simulink model "BATTERY_PV_IMPLEMENTATION"  (R2024a)
settings: Solver=VariableStepAuto  StartTime=0.0  StopTime=0.23  RelTol=1e-3
values from neighbouring files (symbols this model uses):
  a = 1.3    [TEST.m]    (also in batter_y.m = -k_omega / J)
  beta = [0.0000, 0.0306, 0.0560, 0.0772, 0.0953, 0.1113, 0.1254, 0.1382,          0.1499, 0.1607, 0.1783, 0.2134, 0.2421, 0.2669, 0.2890, 0.3091,          0.3279, 0.3456, 0.3625, 0.3789]'    [batter_y.m]
  Cdc = 278e-3    (= 0.278)    [TEST.m]    (also in batter_y.m)
  Clink = 2 * (3 / 4) * (Pnom / Fnom * 2 / Vnom_dc^2)    (= 0.325520833333)    [batter_y.m]
  fg = 60    [TEST.m]    (also in batter_y.m)
  Fnom = 60    [batter_y.m]
  Gn = 1000    [TEST.m]    (also in batter_y.m)
  Ipv_n = Isc_n*(Rp+Rs)/Rp    (= 8.21426513558)    [TEST.m]    (also in batter_y.m)
  Isc_n = 8.21    [TEST.m]    (also in batter_y.m)
  k = 1.3806503e-23    [TEST.m]    (also in batter_y.m)
  k_I = a./(b.*tau_ref)    [batter_y.m]
  k_P = 5./(b.*tau_ref)    [batter_y.m]
  KI = 0.0032    [TEST.m]    (also in batter_y.m)
  Ki_C = Rc/tau_C    (= 0.768)    [TEST.m]    (also in batter_y.m)
  Ki_DC = omega_DC^2*Cdc    [TEST.m]    (also in batter_y.m)
  Ki_Ireg = 20    [batter_y.m]
  Ki_P = 1/(Ki_pq*tau_P)    [TEST.m]    (also in batter_y.m)
  Ki_PLL = Kp_PLL/tau_PLL    [TEST.m]    (also in batter_y.m)
  Kp_C = Lc/tau_C    (= 0.020372)    [TEST.m]    (also in batter_y.m)
  Kp_DC = 2*xi_DC*omega_DC*Cdc    [TEST.m]    (also in batter_y.m)
  Kp_Ireg = 0.3    [batter_y.m]
  Kp_P = tau_C/(Ki_pq*tau_P)    [TEST.m]    (also in batter_y.m)
  Kp_PLL = xi_PLL*2*omega_PLL/Vp    [TEST.m]    (also in batter_y.m)
  KV = -0.123    [TEST.m]    (also in batter_y.m)
  KVmp = Vmp_n/Voc_n    (= 0.799392097264)    [TEST.m]    (also in batter_y.m)
  Lc = 20.372e-6    (= 2.0372e-05)    [TEST.m]    (also in batter_y.m)
  Lchoke = 0.15    [batter_y.m]
  Ltot_pu = Lxf + Lchoke    (= 0.21)    [batter_y.m]
  Lxf = TotalLeakage    (= 0.06)    [batter_y.m]
  Np = 345    [TEST.m]    (also in batter_y.m)
  Ns = 45    [TEST.m]    (also in batter_y.m)
  Ns_cell = 54    [TEST.m]    (also in batter_y.m)
  Pnom = PnomkW*1e3    (= 500000)    [TEST.m]    (also in batter_y.m = 1500000)
  q = 1.6021764e-19    [TEST.m]    (also in batter_y.m)
  Rc = 0.768e-3    (= 0.000768)    [TEST.m]    (also in batter_y.m)
  Rchoke = 0.15 / 100    (= 0.0015)    [batter_y.m]
  Rp = 425.405    [TEST.m]    (also in batter_y.m)
  Rs = 0.221    [TEST.m]    (also in batter_y.m)
  Rtot_pu = Rxf + Rchoke    (= 0.0039)    [batter_y.m]
  Rxf = TotalLeakage / 25    (= 0.0024)    [batter_y.m]
  Tn = 25    [TEST.m]    (also in batter_y.m)
  Ts = 5e-5    (= 5e-05)    [TEST.m]    (also in batter_y.m)
  Ts_Control = 5e-5    (= 5e-05)    [TEST.m]    (also in batter_y.m)
  v = [11.2600, 11.5378, 11.8156, 12.0933, 12.3711, 12.6489, 12.9267,       13.2044, 13.4822, 13.7600, 14.2600, 15.4533, 16.6467, 17.8400,       19.0333, 20.2267, 21.4200, 22.6133, 23.8067, 25.0000]'    [batter_y.m]
  Vdc = 1200    [TEST.m]    (also in batter_y.m)
  Vnom_dc = 480    [batter_y.m]
  Vnom_prim = 2400    [batter_y.m]
  Vnom_sec = 0.85 * Vnom_dc / 2 / sqrt(2) * sqrt(3)    [batter_y.m]
  Voc_n = 32.9    [TEST.m]    (also in batter_y.m)
  Vp = Ug*sqrt(2)/sqrt(3)    [TEST.m]    (also in batter_y.m)
  Zbase = Vnom_sec^2 / Pnom    [batter_y.m]
undefined symbols (not defined in the file or in its folder): D1, Delta, Ion, Lithium, para_mdl
libraries: spsSeriesRLCBranchLib x25, slpidlib x11, spsThreePhaseSeriesRLCLoadLib x9, spsThreePhaseVIMeasurementLib x7, spsSeriesRLCLoadLib x5, spsGroundLib x5, spsThreePhaseTransformerTwoWindingsLib x5, spsabctodq0Lib x4, spsControlledVoltageSourceLib x3, spsPower3phInstantaneousLib x3, spsCurrentMeasurementLib x2, spsControlledCurrentSourceLib x2
(part 3 of 3)

== system BATTERY_PV_IMPLEMENTATION/Subsystem2/Current Control/Current Regulator ==
  note: Id positive --> The converter generates active power ("Inverter mode") = Active Power P positive
  note: Iq positive --> The converter absorbs reactive power ("Inductive mode") = Reactive Power Q negative
  note: Sign Convention: Current going out of the converter = positive current
  note: Current Regulator
      | ================
  VdVq_meas : Inport  PortDimensions=2
  IdIq_meas : Inport  Port=2  PortDimensions=2
  IdIq_ref : Inport  Port=3  PortDimensions=2
  Add1 : Sum  Inputs=++-
  Add2 : Sum
  Add3 : Sum  Inputs=+++
  Demux : Demux  Outputs=2
  Demux1 : Demux  Outputs=2
  Lff : Gain  Gain=Ltot_pu  SaturateOnIntegerOverflow=on  OutDataTypeStr=Inherit: Same as input  ParamDataTypeStr=Inherit: Same as input
  "Lff  " : Gain  Gain=Ltot_pu  SaturateOnIntegerOverflow=on  OutDataTypeStr=Inherit: Same as input  ParamDataTypeStr=Inherit: Same as input
  Mux : Mux  Inputs=2
  PI : slpidlib/PID Controller  Controller=PI  Form=Parallel  TimeDomain=Discrete-time  UseExternalTs=off  SampleTime=Ts_Control  IntegratorMethod=Forward Euler  FilterMethod=Forward Euler  ControllerParametersSource=internal  P=Kp_Ireg  I=Ki_Ireg  UseKiTs=off  D=0  UseExternalDerivativeSource=off  N=100  UseFilter=on  TunerSelectOption=Transfer Function Based (PID Tuner App)  InitialConditionSource=internal  InitialConditionForIntegrator=0  InitialConditionForFilter=0  DifferentiatorICPrevScaledInput=0  ExternalReset=none  TrackingMode=off  Kt=1  LimitOutput=on  SatLimitsSource=internal  UpperSaturationLimit=1.5  LowerSaturationLimit=-1.5  LinearizeAsGain=off  AntiWindupMode=clamping  Kb=1  LimitIntegrator=off  UpperIntegratorSaturationLimit=inf  LowerIntegratorSaturationLimit=-inf  POutMin=[]  POutMax=[]  IOutMin=[]  IOutMax=[]  DOutMin=[]  DOutMax=[]  NOutMin=[]  NOutMax=[]  SumOutMin=[]  SumOutMax=[]  SaturationOutMin=[]  SaturationOutMax=[]  PParamMin=[]  PParamMax=[]  IParamMin=[]  IParamMax=[]  DParamMin=[]  DParamMax=[]  NParamMin=[]  NParamMax=[]  KbParamMin=[]  KbParamMax=[]  KtParamMin=[]  KtParamMax=[]  KbOutMin=[]  KbOutMax=[]  KtOutMin=[]  KtOutMax=[]  IntegratorOutMin=[]  IntegratorOutMax=[]  FilterOutMin=[]  FilterOutMax=[]  SumI1OutMin=[]  SumI1OutMax=[]  SumI2OutMin=[]  SumI2OutMax=[]  SumI3OutMin=[]  SumI3OutMax=[]  SumI4OutMin=[]  SumI4OutMax=[]  SumDOutMin=[]  SumDOutMax=[]  DifferentiatorOutMin=[]  DifferentiatorOutMax=[]  FilterDiffOutCoefMin=[]  FilterDiffOutCoefMax=[]  ReciprocalOutMin=[]  ReciprocalOutMax=[]  SumDenOutMin=[]  SumDenOutMax=[]  SumNumOutMin=[]  SumNumOutMax=[]  DivideOutMin=[]  DivideOutMax=[]  UdiffTsProdOutMin=[]  UdiffTsProdOutMax=[]  NTsProdOutMin=[]  NTsProdOutMax=[]  UintegralTsProdOutMin=[]  UintegralTsProdOutMax=[]  UngainTsProdOutMin=[]  UngainTsProdOutMax=[]  ClampingZeroOutDataTypeStr=Inherit: Inherit via back propagation  ClampingZeroOutMin=[]  ClampingZeroOutMax=[]  FilterDenConstantOutDataTypeStr=Inherit: Inherit via back propagation  FilterDenConstantOutMin=[]  FilterDenConstantOutMax=[]  PCopyOutDataTypeStr=Inherit: Inherit via back propagation  PCopyOutMin=[]  PCopyOutMax=[]  NCopyOutDataTypeStr=Inherit: Inherit via back propagation  NCopyOutMin=[]  NCopyOutMax=[]  IntegratorContinuousStateAttributes=''  IntegratorStateMustResolveToSignalObject=off  IntegratorRTWStateStorageClass=Auto  FilterContinuousStateAttributes=''  FilterStateMustResolveToSignalObject=off  FilterRTWStateStorageClass=Auto  ParallelPVariant=InternalParameters  IdealPVariant=Disabled  IVariant=InternalParameters  DVariant=Disabled  IntegratorVariant=Discrete  SatVariant=Enabled  AWVariant=DiscClampingParallel  PCopyVariant=Disabled  TRVariant=Disabled  FdbkBlocksVariant=Forward  IdealPFdbkVariant=Disabled  SatFdbkVariant=Disabled  DerivativeFilterVariant=Disabled  NVariant=Disabled  NCopyVariant=Disabled_SignalSpec  FilterICVariant=Disabled  IntegratorICVariant=InternalICs  ExternalResetVariant=Disabled  TRSumVariant=Passthrough  SumFdbkVariant=Disabled  SumVariant=Sum_PI  TsampFilterVariant=InternalTs  TsampNgainVariant=Passthrough  TsampIntegralVariant=Disabled_SignalSpec  ExternalSaturationOutDataTypeStr=Inherit: Same as second input  DerivativeSourceVariant=Disabled
  Rff : Gain  Gain=Rtot_pu  SaturateOnIntegerOverflow=on  OutDataTypeStr=Inherit: Same as input  ParamDataTypeStr=Inherit: Same as input
  "Rff " : Gain  Gain=Rtot_pu  SaturateOnIntegerOverflow=on  OutDataTypeStr=Inherit: Same as input  ParamDataTypeStr=Inherit: Same as input
  Saturation : Saturate  UpperLimit=1.5  LowerLimit=-1.5
  Scope : Scope  NumInputPorts=2
  Sum : Sum  Inputs=|-+
  VdVq_conv : Outport  VectorParamsAs1DForOutWhenUnconnected=off
  wires:
  Add3/1 -> Mux/2
  Demux/2 -> Add3/1
  Add1/1 -> Mux/1  "Feedforward"
  Lff/1 -> Add3/3
  Rff/1 -> Add3/2
  Demux1/2 -> Rff/1, "Lff  "/1
  "Lff  "/1 -> Add1/3
  Demux1/1 -> Lff/1, "Rff "/1
  "Rff "/1 -> Add1/2
  Demux/1 -> Add1/1
  VdVq_meas/1 -> Demux/1
  Saturation/1 -> VdVq_conv/1
  Add2/1 -> Saturation/1
  IdIq_meas/1 -> Sum/1
  IdIq_ref/1 -> Demux1/1, Sum/2
  Sum/1 -> PI/1, Scope/1
  PI/1 -> Add2/1, Scope/2  "PI"
  Mux/1 -> Add2/2

== system BATTERY_PV_IMPLEMENTATION/Subsystem2/Current Control/Uabc_ref Generation max (m) = 1 ==
  note: Uref Generation
      | ==============
  note: (Correction for delai of Ts_Control)
  note: (Correction for transformer
      |  D1 connection)
  wt : Inport
  VdVq_conv : Inport  Port=2
  Add1 : Sum  Inputs=++++
  Add2 : Sum
  Complex to Magnitude-Angle : ComplexToMagnitudeAngle
  Constant : Constant  Value=-pi/6
  Constant1 : Constant  Value=Vnom_dc
  Constant2 : Constant  Value="[ 0  -2*pi/3  2*pi/3  ]"
  Constant3 : Constant  Value=Vnom_sec*sqrt(2)/sqrt(3)
  Constant4 : Constant  Value=Ts_Control*Fnom*(2*pi)
  Demux1 : Demux  Outputs=2
  Gain1 : Gain  Gain=1/2
  Product : Product  Inputs=*/  RndMeth=Zero
  Product1 : Product  Inputs=*/  RndMeth=Zero
  Product2 : Product  Inputs=**  RndMeth=Zero
  Real-Imag to Complex : RealImagToComplex
  Trigonometric Function : Trigonometry
  Uabc_ref : Outport  VectorParamsAs1DForOutWhenUnconnected=off
  wires:
  Constant4/1 -> Add1/4
  wt/1 -> Add1/1
  Product2/1 -> Uabc_ref/1
  Trigonometric Function/1 -> Product2/2
  Complex to Magnitude-Angle/1 -> Product2/1
  Add2/1 -> Trigonometric Function/1
  Add1/1 -> Add2/2
  Complex to Magnitude-Angle/2 -> Add2/1
  Product/1 -> Product1/2
  Constant3/1 -> Product/2
  Constant/1 -> Add1/3
  Constant2/1 -> Add1/2
  Demux1/2 -> Real-Imag to Complex/2
  Demux1/1 -> Real-Imag to Complex/1
  Real-Imag to Complex/1 -> Complex to Magnitude-Angle/1
  Gain1/1 -> Product/1
  Product1/1 -> Demux1/1
  VdVq_conv/1 -> Product1/1
  Constant1/1 -> Gain1/1

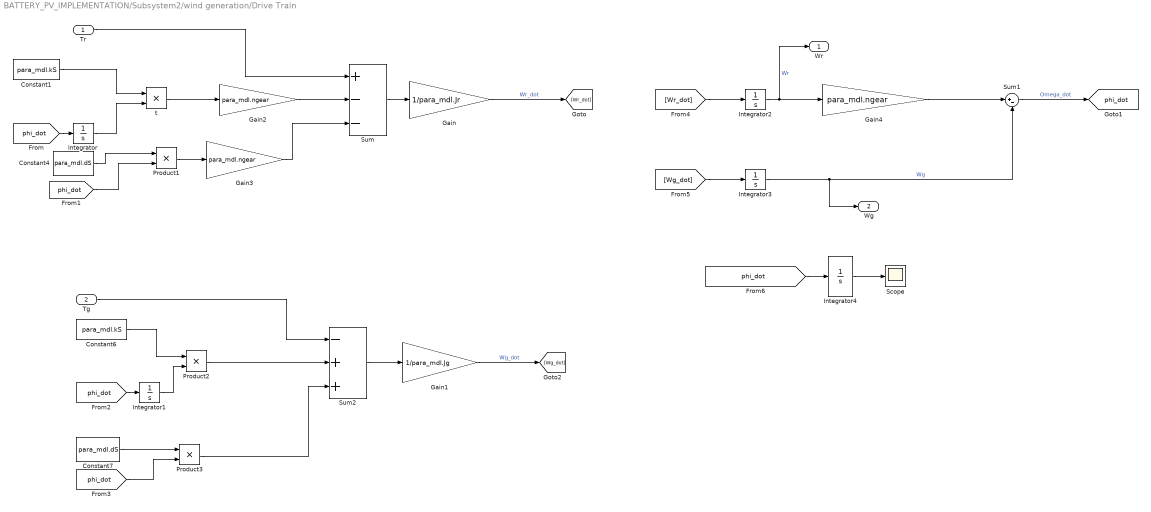
== system BATTERY_PV_IMPLEMENTATION/Subsystem2/wind generation/Drive Train ==
  Tr : Inport
  Tg : Inport  Port=2
  Constant1 : Constant  Value=para_mdl.kS
  Constant4 : Constant  Value=para_mdl.dS
  Constant6 : Constant  Value=para_mdl.kS
  Constant7 : Constant  Value=para_mdl.dS
  Gain : Gain  Gain=1/para_mdl.Jr
  Gain1 : Gain  Gain=1/para_mdl.Jg
  Gain2 : Gain  Gain=para_mdl.ngear
  Gain3 : Gain  Gain=para_mdl.ngear
  Gain4 : Gain  Gain=para_mdl.ngear
  Integrator{,1..4} (5 alike) : Integrator
  Product1 : Product
  Product2 : Product
  Product3 : Product
  Scope : Scope
  Sum : Sum  Inputs=+--
  Sum1 : Sum  Inputs=|+-
  Sum2 : Sum  Inputs=-++
  t : Product
  Wr : Outport
  Wg : Outport  Port=2
  tag scope: phi_dot=global
  wires:
  Product1/1 -> Gain3/1
  Integrator4/1 -> Scope/1
  [phi_dot] -> Integrator4/1
  Gain3/1 -> Sum/3
  Gain2/1 -> Sum/2
  Product3/1 -> Sum2/3
  Product2/1 -> Sum2/2
  t/1 -> Gain2/1
  Tr/1 -> Sum/1
  Gain/1 -> [Wr_dot]  "Wr_dot"
  [Wg_dot] -> Integrator3/1
  Integrator/1 -> t/2
  Integrator1/1 -> Product2/2
  [phi_dot] -> Integrator/1
  [phi_dot] -> Product1/2
  Constant1/1 -> t/1
  Gain1/1 -> [Wg_dot]  "Wg_dot"
  [phi_dot] -> Product3/2
  Sum2/1 -> Gain1/1
  Sum/1 -> Gain/1
  Integrator3/1 -> Sum1/2, Wg/1  "Wg"
  Constant7/1 -> Product3/1
  Sum1/1 -> [phi_dot]  "Omega_dot"
  Tg/1 -> Sum2/1
  Constant6/1 -> Product2/1
  Integrator2/1 -> Gain4/1, Wr/1  "Wr"
  Constant4/1 -> Product1/1
  [phi_dot] -> Integrator1/1
  Gain4/1 -> Sum1/1
  [Wr_dot] -> Integrator2/1

== system BATTERY_PV_IMPLEMENTATION/Subsystem2/wind generation/If Action Subsystem ==
  omega_r : Inport
  Wind Speed : Inport  Port=2
  Action Port : ActionPort  ActionPortLabel=else
  Add : Sum  Inputs=-+
  Constant : Constant  Value=para_mdl.omega_r_R
  Integrator1 : Integrator
  KI1 : Display
  KP1 : Display
  Product : Product
  Product1 : Product
  Scope6 : Scope  NumInputPorts=2
  Subsystem1 : Subsystem  Priority=1
  Sum1 : Sum  Inputs=|++
  Beta_1 : Outport
  wires:
  Product1/1 -> Sum1/2
  omega_r/1 -> Add/1
  Subsystem1/1(" KP") -> Product/1, KP1/1, Scope6/1
  Subsystem1/2(" KI") -> KI1/1, Product1/2, Scope6/2
  Sum1/1 -> Beta_1/1
  Wind Speed/1 -> Subsystem1/1(Speed)
  Product/1 -> Sum1/1
  Add/1 -> Product/2, Integrator1/1
  Integrator1/1 -> Product1/1
  Constant/1 -> Add/2

== system BATTERY_PV_IMPLEMENTATION/Subsystem2/wind generation/If Action Subsystem1 ==
  Input : Inport
  Input1 : Inport  Port=2
  Action Port : ActionPort  ActionPortLabel=if(u1 ~= 3)
  MATLAB Function1 : MATLAB Function  TreatAsAtomicUnit=on
  Output : Outport
  wires:
  MATLAB Function1/1(Tg) -> Output/1
  Input/1 -> MATLAB Function1/1(wg)
  Input1/1 -> MATLAB Function1/2(region)

== system BATTERY_PV_IMPLEMENTATION/Subsystem2/wind generation/Subsystem ==
  Lamda : Inport
  Beta : Inport  Port=2
  2-D Lookup Table : Lookup_n-D  BreakpointsForDimension1=para_mdl.CQ_lambdas  BreakpointsForDimension2=para_mdl.CQ_betas  Table=para_mdl.CQ_entries  InternalRulePriority=Speed  RndMeth=Simplest
      settings: InputPortMap=u0,u1
  2-D Lookup Table1 : Lookup_n-D  BreakpointsForDimension1=para_mdl.CT_lambdas  BreakpointsForDimension2=para_mdl.CT_betas  Table=para_mdl.CT_entries  InternalRulePriority=Speed  RndMeth=Simplest
      settings: InputPortMap=u0,u1
  CQ : Outport
  CT : Outport  Port=2
  wires:
  2-D Lookup Table/1 -> CQ/1
  Lamda/1 -> 2-D Lookup Table/1, 2-D Lookup Table1/1
  2-D Lookup Table1/1 -> CT/1
  Beta/1 -> 2-D Lookup Table1/2, 2-D Lookup Table/2

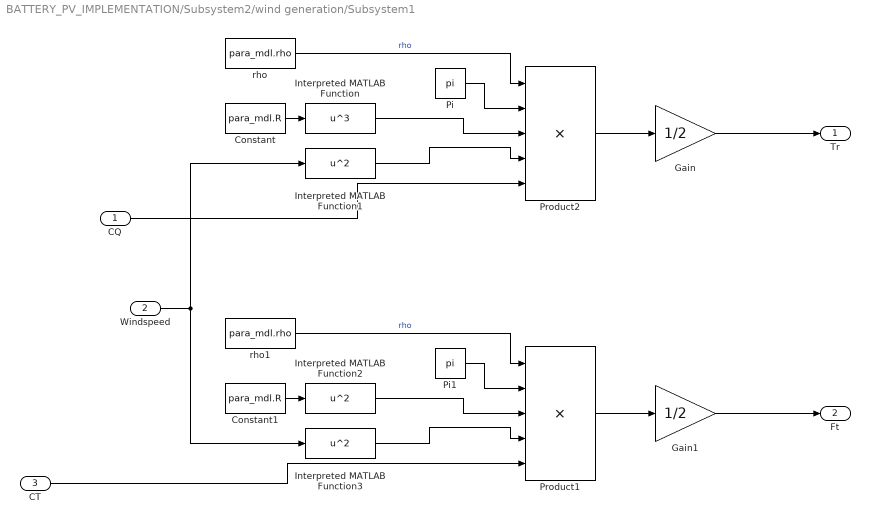
== system BATTERY_PV_IMPLEMENTATION/Subsystem2/wind generation/Subsystem1 ==
  CQ : Inport
  Windspeed : Inport  Port=2
  CT : Inport  Port=3
  Constant : Constant  Value=para_mdl.R
  Constant1 : Constant  Value=para_mdl.R
  Gain : Gain  Gain=1/2
  Gain1 : Gain  Gain=1/2
  Interpreted MATLAB Function : MATLABFcn  MATLABFcn=u^3
  Interpreted MATLAB Function1 : MATLABFcn  MATLABFcn=u^2
  Interpreted MATLAB Function2 : MATLABFcn  MATLABFcn=u^2
  Interpreted MATLAB Function3 : MATLABFcn  MATLABFcn=u^2
  Pi : Constant  Value=pi  OutDataTypeStr=Inherit: Inherit via back propagation
  Pi1 : Constant  Value=pi  OutDataTypeStr=Inherit: Inherit via back propagation
  Product1 : Product  Inputs=5
  Product2 : Product  Inputs=5
  rho : Constant  Value=para_mdl.rho
  rho1 : Constant  Value=para_mdl.rho
  Tr : Outport
  Ft : Outport  Port=2
  wires:
  CT/1 -> Product1/5
  CQ/1 -> Product2/5
  rho1/1 -> Product1/1  "rho"
  Interpreted MATLAB Function/1 -> Product2/3
  rho/1 -> Product2/1  "rho"
  Interpreted MATLAB Function2/1 -> Product1/3
  Constant1/1 -> Interpreted MATLAB Function2/1
  Gain1/1 -> Ft/1
  Constant/1 -> Interpreted MATLAB Function/1
  Gain/1 -> Tr/1
  Interpreted MATLAB Function3/1 -> Product1/4
  Pi1/1 -> Product1/2
  Interpreted MATLAB Function1/1 -> Product2/4
  Pi/1 -> Product2/2
  Product1/1 -> Gain1/1
  Windspeed/1 -> Interpreted MATLAB Function3/1, Interpreted MATLAB Function1/1
  Product2/1 -> Gain/1

== system BATTERY_PV_IMPLEMENTATION/Subsystem2/wind generation/Subsystem2 ==
  wg : Inport
  Tg : Inport  Port=2
  MATLAB Function : MATLAB Function  TreatAsAtomicUnit=on
  turbineRegion : Outport
  wires:
  MATLAB Function/1(turbineRegion) -> turbineRegion/1
  Tg/1 -> MATLAB Function/2(Tg)
  wg/1 -> MATLAB Function/1(wg)

== system BATTERY_PV_IMPLEMENTATION/Controlled PV Array/VSC Control/Current Control/Inverse Park Transformation ==
  qd0 : Inport
  theta : Inport  Port=2
  Constant2 : Constant
  Constant3 : Constant  Value=2*pi/3
  Cos : Trigonometry  Operator=cos
  Matrix Concatenate : Concatenate  NumInputs=3  Mode=Multidimensional array  ConcatenateDimension=2
  Matrix Multiply : Product  Multiplication=Matrix(*)
  Mux1 : Mux  Inputs=3
  Mux2 : Mux  Inputs=3
  Sin : Trigonometry
  Sum : Sum  Inputs=+-|
  Sum1 : Sum  Inputs=++|
  abc : Outport
  wires:
  Constant3/1 -> Sum/2, Sum1/2
  theta/1 -> Mux1/1, Sum1/1, Sum/1
  qd0/1 -> Matrix Multiply/2
  Sum/1 -> Mux1/2
  Sum1/1 -> Mux1/3
  Matrix Multiply/1 -> abc/1
  Mux2/1 -> Matrix Concatenate/3
  Matrix Concatenate/1 -> Matrix Multiply/1
  Mux1/1 -> Cos/1, Sin/1
  Cos/1 -> Matrix Concatenate/1
  Constant2/1 -> Mux2/2, Mux2/3, Mux2/1
  Sin/1 -> Matrix Concatenate/2

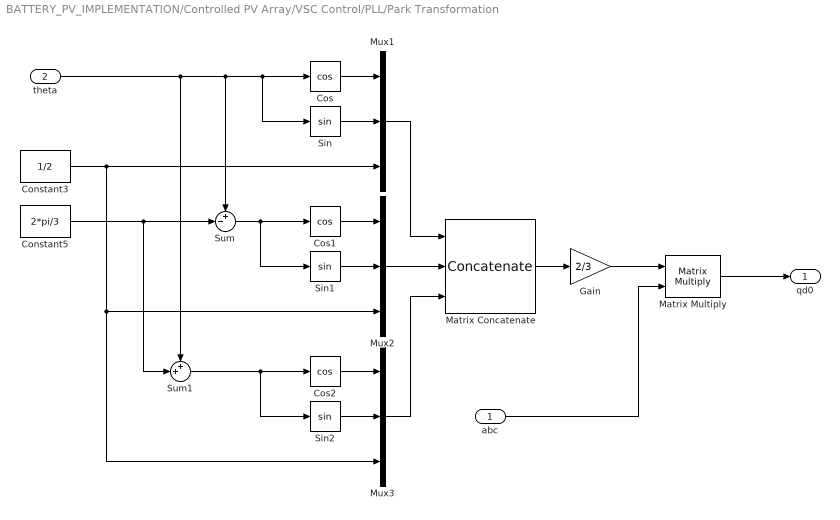
== system BATTERY_PV_IMPLEMENTATION/Controlled PV Array/VSC Control/PLL/Park Transformation ==
  abc : Inport
  theta : Inport  Port=2
  Constant3 : Constant  Value=1/2
  Constant5 : Constant  Value=2*pi/3
  Cos : Trigonometry  Operator=cos
  Cos1 : Trigonometry  Operator=cos
  Cos2 : Trigonometry  Operator=cos
  Gain : Gain  Gain=2/3
  Matrix Concatenate : Concatenate  NumInputs=3  Mode=Multidimensional array  ConcatenateDimension=2
  Matrix Multiply : Product  Multiplication=Matrix(*)
  Mux1 : Mux  Inputs=3
  Mux2 : Mux  Inputs=3
  Mux3 : Mux  Inputs=3
  Sin : Trigonometry
  Sin1 : Trigonometry
  Sin2 : Trigonometry
  Sum : Sum  Inputs=+-|
  Sum1 : Sum  Inputs=++|
  qd0 : Outport
  wires:
  Constant5/1 -> Sum1/2, Sum/2
  Matrix Multiply/1 -> qd0/1
  Matrix Concatenate/1 -> Gain/1
  Sin1/1 -> Mux2/2
  Mux3/1 -> Matrix Concatenate/3
  Cos1/1 -> Mux2/1
  Mux1/1 -> Matrix Concatenate/1
  Cos2/1 -> Mux3/1
  Sum/1 -> Cos1/1, Sin1/1
  Mux2/1 -> Matrix Concatenate/2
  Sin/1 -> Mux1/2
  Sin2/1 -> Mux3/2
  Constant3/1 -> Mux1/3, Mux2/3, Mux3/3
  theta/1 -> Sin/1, Cos/1, Sum/1, Sum1/1
  Gain/1 -> Matrix Multiply/1
  Cos/1 -> Mux1/1
  abc/1 -> Matrix Multiply/2
  Sum1/1 -> Cos2/1, Sin2/1

== system BATTERY_PV_IMPLEMENTATION/Subsystem/Inverter Control/Current Control/Current Regulator ==
  note: Current Regulator
      | ================
  note: Sign Convention: Current going out of the converter = positive current
  note: Iq positive --> The converter absorbs reactive power ("Inductive mode") = Reactive Power Q negative
  note: Id positive --> The converter generates active power ("Inverter mode") = Active Power P positive
  VdVq_meas : Inport  PortDimensions=2
  IdIq_meas : Inport  Port=2  PortDimensions=2
  IdIq_ref : Inport  Port=3  PortDimensions=2
  Add1 : Sum  Inputs=++-
  Add2 : Sum
  Add3 : Sum  Inputs=+++
  Demux : Demux  Outputs=2
  Demux1 : Demux  Outputs=2
  Lff : Gain  Gain=Ltot_pu  SaturateOnIntegerOverflow=on  OutDataTypeStr=Inherit: Same as input  ParamDataTypeStr=Inherit: Same as input
  "Lff  " : Gain  Gain=Ltot_pu  SaturateOnIntegerOverflow=on  OutDataTypeStr=Inherit: Same as input  ParamDataTypeStr=Inherit: Same as input
  Mux : Mux  Inputs=2
  PI : slpidlib/PID Controller  Controller=PI  Form=Parallel  TimeDomain=Discrete-time  UseExternalTs=off  SampleTime=Ts_Control  IntegratorMethod=Forward Euler  FilterMethod=Forward Euler  ControllerParametersSource=internal  P=Kp_Ireg  I=Ki_Ireg  UseKiTs=off  D=0  UseExternalDerivativeSource=off  N=100  UseFilter=on  TunerSelectOption=Transfer Function Based (PID Tuner App)  InitialConditionSource=internal  InitialConditionForIntegrator=0  InitialConditionForFilter=0  DifferentiatorICPrevScaledInput=0  ExternalReset=none  TrackingMode=off  Kt=1  LimitOutput=on  SatLimitsSource=internal  UpperSaturationLimit=1.5  LowerSaturationLimit=-1.5  LinearizeAsGain=off  AntiWindupMode=clamping  Kb=1  LimitIntegrator=off  UpperIntegratorSaturationLimit=inf  LowerIntegratorSaturationLimit=-inf  POutMin=[]  POutMax=[]  IOutMin=[]  IOutMax=[]  DOutMin=[]  DOutMax=[]  NOutMin=[]  NOutMax=[]  SumOutMin=[]  SumOutMax=[]  SaturationOutMin=[]  SaturationOutMax=[]  PParamMin=[]  PParamMax=[]  IParamMin=[]  IParamMax=[]  DParamMin=[]  DParamMax=[]  NParamMin=[]  NParamMax=[]  KbParamMin=[]  KbParamMax=[]  KtParamMin=[]  KtParamMax=[]  KbOutMin=[]  KbOutMax=[]  KtOutMin=[]  KtOutMax=[]  IntegratorOutMin=[]  IntegratorOutMax=[]  FilterOutMin=[]  FilterOutMax=[]  SumI1OutMin=[]  SumI1OutMax=[]  SumI2OutMin=[]  SumI2OutMax=[]  SumI3OutMin=[]  SumI3OutMax=[]  SumI4OutMin=[]  SumI4OutMax=[]  SumDOutMin=[]  SumDOutMax=[]  DifferentiatorOutMin=[]  DifferentiatorOutMax=[]  FilterDiffOutCoefMin=[]  FilterDiffOutCoefMax=[]  ReciprocalOutMin=[]  ReciprocalOutMax=[]  SumDenOutMin=[]  SumDenOutMax=[]  SumNumOutMin=[]  SumNumOutMax=[]  DivideOutMin=[]  DivideOutMax=[]  UdiffTsProdOutMin=[]  UdiffTsProdOutMax=[]  NTsProdOutMin=[]  NTsProdOutMax=[]  UintegralTsProdOutMin=[]  UintegralTsProdOutMax=[]  UngainTsProdOutMin=[]  UngainTsProdOutMax=[]  ClampingZeroOutDataTypeStr=Inherit: Inherit via back propagation  ClampingZeroOutMin=[]  ClampingZeroOutMax=[]  FilterDenConstantOutDataTypeStr=Inherit: Inherit via back propagation  FilterDenConstantOutMin=[]  FilterDenConstantOutMax=[]  PCopyOutDataTypeStr=Inherit: Inherit via back propagation  PCopyOutMin=[]  PCopyOutMax=[]  NCopyOutDataTypeStr=Inherit: Inherit via back propagation  NCopyOutMin=[]  NCopyOutMax=[]  IntegratorContinuousStateAttributes=''  IntegratorStateMustResolveToSignalObject=off  IntegratorRTWStateStorageClass=Auto  FilterContinuousStateAttributes=''  FilterStateMustResolveToSignalObject=off  FilterRTWStateStorageClass=Auto  ParallelPVariant=InternalParameters  IdealPVariant=Disabled  IVariant=InternalParameters  DVariant=Disabled  IntegratorVariant=Discrete  SatVariant=Enabled  AWVariant=DiscClampingParallel  PCopyVariant=Disabled  TRVariant=Disabled  FdbkBlocksVariant=Forward  IdealPFdbkVariant=Disabled  SatFdbkVariant=Disabled  DerivativeFilterVariant=Disabled  NVariant=Disabled  NCopyVariant=Disabled_SignalSpec  FilterICVariant=Disabled  IntegratorICVariant=InternalICs  ExternalResetVariant=Disabled  TRSumVariant=Passthrough  SumFdbkVariant=Disabled  SumVariant=Sum_PI  TsampFilterVariant=InternalTs  TsampNgainVariant=Passthrough  TsampIntegralVariant=Disabled_SignalSpec  ExternalSaturationOutDataTypeStr=Inherit: Same as second input  DerivativeSourceVariant=Disabled
  Rff : Gain  Gain=Rtot_pu  SaturateOnIntegerOverflow=on  OutDataTypeStr=Inherit: Same as input  ParamDataTypeStr=Inherit: Same as input
  "Rff " : Gain  Gain=Rtot_pu  SaturateOnIntegerOverflow=on  OutDataTypeStr=Inherit: Same as input  ParamDataTypeStr=Inherit: Same as input
  Saturation : Saturate  UpperLimit=1.5  LowerLimit=-1.5
  Scope : Scope  NumInputPorts=2
  Sum : Sum  Inputs=|-+
  VdVq_conv : Outport  VectorParamsAs1DForOutWhenUnconnected=off
  wires:
  Mux/1 -> Add2/2
  PI/1 -> Scope/2, Add2/1  "PI"
  Sum/1 -> Scope/1, PI/1
  IdIq_ref/1 -> Sum/2, Demux1/1
  IdIq_meas/1 -> Sum/1
  Add2/1 -> Saturation/1
  Saturation/1 -> VdVq_conv/1
  VdVq_meas/1 -> Demux/1
  Demux/1 -> Add1/1
  "Rff "/1 -> Add1/2
  Demux1/1 -> "Rff "/1, Lff/1
  "Lff  "/1 -> Add1/3
  Demux1/2 -> "Lff  "/1, Rff/1
  Rff/1 -> Add3/2
  Lff/1 -> Add3/3
  Add1/1 -> Mux/1  "Feedforward"
  Demux/2 -> Add3/1
  Add3/1 -> Mux/2

== system BATTERY_PV_IMPLEMENTATION/Subsystem/Inverter Control/Current Control/Uabc_ref Generation max (m) = 1 ==
  note: (Correction for transformer
      |  D1 connection)
  note: (Correction for delai of Ts_Control)
  note: Uref Generation
      | ==============
  wt : Inport
  VdVq_conv : Inport  Port=2
  Add1 : Sum  Inputs=++++
  Add2 : Sum
  Complex to Magnitude-Angle : ComplexToMagnitudeAngle
  Constant : Constant  Value=-pi/6
  Constant1 : Constant  Value=Vnom_dc
  Constant2 : Constant  Value="[ 0  -2*pi/3  2*pi/3  ]"
  Constant3 : Constant  Value=Vnom_sec*sqrt(2)/sqrt(3)
  Constant4 : Constant  Value=Ts_Control*Fnom*(2*pi)
  Demux1 : Demux  Outputs=2
  Gain1 : Gain  Gain=1/2
  Product : Product  Inputs=*/  RndMeth=Zero
  Product1 : Product  Inputs=*/  RndMeth=Zero
  Product2 : Product  Inputs=**  RndMeth=Zero
  Real-Imag to Complex : RealImagToComplex
  Trigonometric Function : Trigonometry
  Uabc_ref : Outport  VectorParamsAs1DForOutWhenUnconnected=off
  wires:
  Constant1/1 -> Gain1/1
  VdVq_conv/1 -> Product1/1
  Product1/1 -> Demux1/1
  Gain1/1 -> Product/1
  Real-Imag to Complex/1 -> Complex to Magnitude-Angle/1
  Demux1/1 -> Real-Imag to Complex/1
  Demux1/2 -> Real-Imag to Complex/2
  Constant2/1 -> Add1/2
  Constant/1 -> Add1/3
  Constant3/1 -> Product/2
  Product/1 -> Product1/2
  Complex to Magnitude-Angle/2 -> Add2/1
  Add1/1 -> Add2/2
  Add2/1 -> Trigonometric Function/1
  Complex to Magnitude-Angle/1 -> Product2/1
  Trigonometric Function/1 -> Product2/2
  Product2/1 -> Uabc_ref/1
  wt/1 -> Add1/1
  Constant4/1 -> Add1/4

== system BATTERY_PV_IMPLEMENTATION/Subsystem2/wind generation/If Action Subsystem/Subsystem1 ==
  Speed : Inport
  2-D Lookup KI1 : Lookup_n-D  NumberOfTableDimensions=1  BreakpointsForDimension1=v  BreakpointsForDimension2=beta  Table=k_I  InternalRulePriority=Speed  RndMeth=Simplest
  2-D Lookup KP1 : Lookup_n-D  NumberOfTableDimensions=1  BreakpointsForDimension1=v  BreakpointsForDimension2=[1:3]  Table=k_P  InternalRulePriority=Speed  RndMeth=Simplest
  Display : Display
  Display1 : Display
  To Workspace : ToWorkspace  VariableName=KP1  SaveFormat=Timeseries  SampleTime=-1
  To Workspace1 : ToWorkspace  VariableName=KI1  SaveFormat=Timeseries  SampleTime=-1
  " KP" : Outport
  " KI" : Outport  Port=2
  wires:
  2-D Lookup KP1/1 -> To Workspace/1, Display/1, " KP"/1
  Speed/1 -> 2-D Lookup KI1/1, 2-D Lookup KP1/1
  2-D Lookup KI1/1 -> To Workspace1/1, Display1/1, " KI"/1

== matlab function BATTERY_PV_IMPLEMENTATION/Subsystem2/wind generation/Subsystem2/MATLAB Function ==
  settings: updateMethod=DISCRETE
  data: wg input; turbineRegion output; Tg input
function turbineRegion = fcn(wg, Tg)
    %#codegen

    % Define the thresholds for the conditions
    wg_rated = 1.229087000000000e+02;
    wg_R1_max = wg_rated * 0.5708; 
    wg_R1_5_max = wg_rated * 0.7421;
    wg_R2_max = wg_rated * 0.9782;
    wg_R2_5_max = wg_rated * 0.99;
     
    dwg = 2;
    Tg_max = 4.309385747306741e+04;

    % Define a persistent variable to store the previous region
    persistent prev_region
    if isempty(prev_region)
        prev_region = 1; % initialize with the starting region
    end
    % Declare that prev_region can have a variable size
    coder.varsize('prev_region', [1, 5], [0, 1]); % [1, 5] is the maximum size, [0, 1] indicates that the second dimension can vary

    % Initialize the region output
    turbineRegion = 0;
    % Check the conditions for each region
    switch prev_region
        case 1 % Region_1
            if wg > wg_R1_max
                turbineRegion = 1.5; % Region_1.5
            else
                turbineRegion = 1; % Region_1
            end
        case 2 % Region_1.5
            if wg > wg_R1_5_max
                turbineRegion = 2; % Region_2
            elseif wg <= wg_R1_max
                turbineRegion = 1; % Region_1
            else
                turbineRegion = 1.5; % Region_1.5
            end
        case 3 % Region_2
            if wg > wg_R2_max && Tg > Tg_max
                turbineRegion = 2.5; % Region_2.5
            elseif wg <= wg_R1_5_max
                turbineRegion = 1.5; % Region_1.5
            else
                turbineRegion = 2; % Region_2
            end
        case 4 % Region_2.5
            if wg > wg_R2_5_max && Tg > Tg_max
                turbineRegion = 3; % Region_3
            elseif wg <= (wg_R2_max - dwg)
                turbineRegion = 2; % Region_2
            else
                turbineRegion = 2.5; % Region_2.5
            end
        case 5 % Region_3
            if wg <= wg_R2_5_max || Tg <= Tg_max
                turbineRegion = 2.5; % Region_2.5
            else
                turbineRegion = 3; % Region_3
            end
    end

    % Update the previous region
    prev_region = find([1, 1.5, 2, 2.5, 3] == turbineRegion);
end

== matlab function BATTERY_PV_IMPLEMENTATION/Subsystem2/wind generation/If Action Subsystem1/MATLAB Function1 ==
  data: wg input; Tg output; region input
function Tg = calculateTg(wg, region)
    % Calculation for Tg based on operating region

    wg_rated = 1.229087000000000e+02;
    Tg_max = 4.309385747306741e+04;
    k_Opt = 2.418610624349642;
    %k_Opt = 0.5 * 1.2250 * pi * 63^5 * (0.4876/(97^3*7.5^3)) * wg^2;
    
    switch region
        case 1
            Tg = 0; % Region 1
        case 1.5
            Tg = (3*(wg/wg_rated) - 1.8)*Tg_max; % Region 1.5
        case 2
            Tg = k_Opt * wg^2; % Region 2
        case 2.5
            Tg = (5.5*(wg/wg_rated) - 4.61)*Tg_max; % Region 2.5
        otherwise
            Tg = 0; % Default value for other regions
    end
end
